simulink model "BO3"  (R2021b)
settings: Solver=VariableStepAuto  StartTime=0.0  StopTime=10.0  RelTol=1e-3
values from neighbouring files (symbols this model uses):
  plant = ss(a,b,c,d)    [demarrage.m]
settings Model: Creator=driss  LastModifiedBy=driss

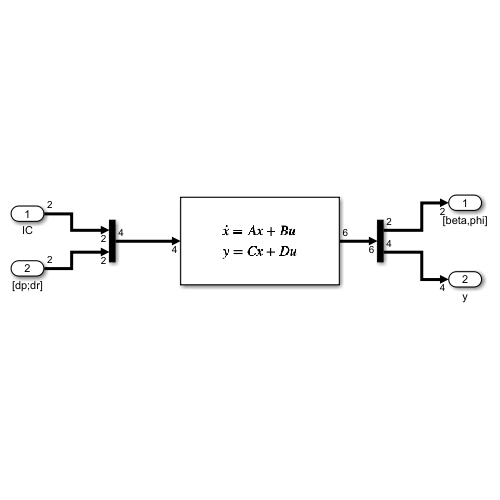
[thumbnail: Simulink's stored preview of the top-level diagram]
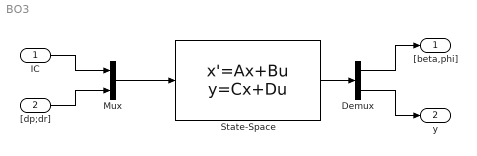
== system BO3 ==
  IC : Inport
  "[dp;dr]" : Inport  Port=2
  Demux : Demux  Outputs=[2 4]
  Mux : Mux  Inputs=[2 2]
  State-Space : StateSpace  A=plant.A  B=[[1 0; 0 0; 0 0 ;0 1] plant.B]  C=[1 0 0 0; 0 0 0 1;plant.C]  D=[zeros(6,2) [zeros(2); plant.D]]  InitialCondition=0
  "[beta,phi]" : Outport
  y : Outport  Port=2
  wires:
  IC/1 -> Mux/1
  "[dp;dr]"/1 -> Mux/2
  Mux/1 -> State-Space/1
  State-Space/1 -> Demux/1
  Demux/2 -> y/1
  Demux/1 -> "[beta,phi]"/1
